simulink model "s20260831_config2torque_sim_chatgpt"  (R2025a)
settings: Solver=daessc  StartTime=0.0  StopTime=inf  FixedStep=0.01  MaxStep=0.01  RelTol=1e-3  AbsTol=1e-3  EnableMultiTasking=on
undefined symbols (not defined in the file or in its folder): X, Y, Z
libraries: sm_lib x8, nesl_utility x3, snake_single_module_library_torque x1, simulink x1, spsSawtoothGeneratorLib x1
settings Model: Creator=dperera  LastModifiedBy=dperera
settings SolverCC: AutoScaleAbsTol=off  AlgebraicLoopSolver=TrustRegion  MaxZcPerStep=1.0
settings DataIOCC: LimitDataPoints=on  MaxDataPoints=10000
settings OptimizationCC: ReuseModelBlockBuffer=off  LifeSpan=inf
settings DebuggingCC: UnconnectedInputMsg=warning  UnconnectedOutputMsg=warning  UnconnectedLineMsg=warning  AllowSymbolicDim=off  SubsystemReferenceDiagnosticForUnitTest=warning  SFUnexpectedBacktrackingDiag=warning  SFNoUnconditionalDefaultTransitionDiag=warning  SFExecutionAtInitializationDiag=none  ArithmeticOperatorsInVariantConditions=warning
settings ModelReferenceCC: EnableRefExpFcnMdlSchedulingChecks=on
settings SFSimCC: SimUseLocalCustomCode=off  CustomCodeUndefinedFunction=UseInterfaceOnly
settings RTWCC: RTWUseLocalCustomCode=off  GPUComputeCapability=3.5  DLArmComputeVersion=19.05
settings CodeAppCC: StateflowObjectComments=on
settings GRTTargetCC: TargetLangStandard=C89/C90 (ANSI)
settings ConfigComp: CovMetricSettings=dw  CovSaveCumulativeToWorkspaceVar=on  CovSaveSingleToWorkspaceVar=on  CovExternalEMLEnable=off  CovSFcnEnable=off
settings SimscapeCC: SimscapeLogType=all  SimscapeLogSimulationStatistics=on  SimscapeLogDataHistory=10000.0

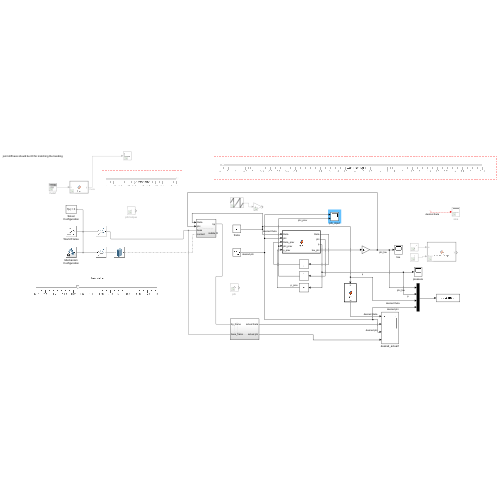
[thumbnail: Simulink's stored preview of the top-level diagram]
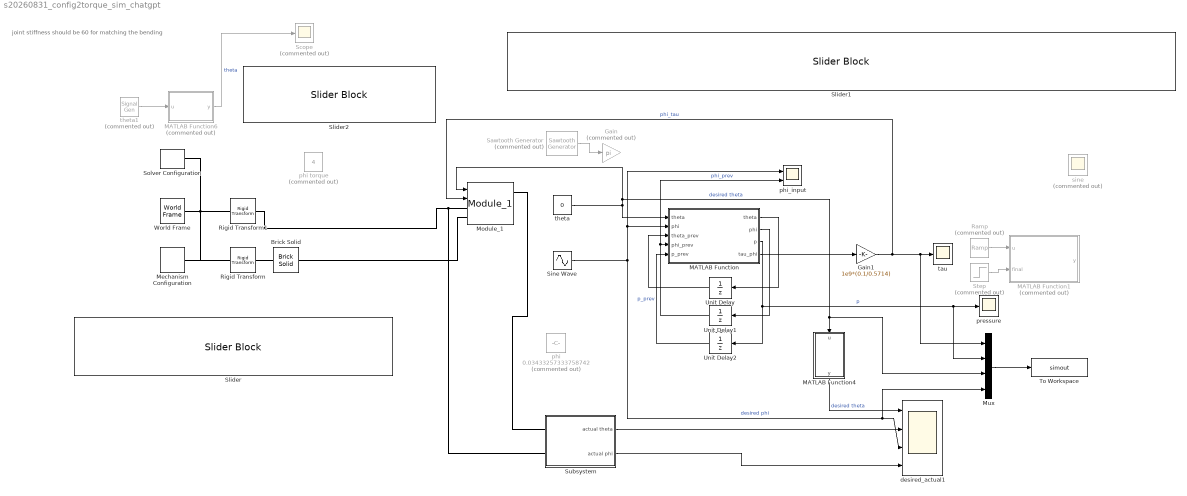
== system s20260831_config2torque_sim_chatgpt ==
  note: joint stiffness should be 60 for matching the bending
  Brick Solid : sm_lib/Body Elements/Brick Solid  BrickDimensions=[0.5 0.5 0.01]  BrickDimensionsUnits=m  ExportEntireGeometry=on  InertiaType=CalculateFromGeometry  BasedOnType=Density  Density=1000  DensityUnits=kg/m^3  Mass=1  MassUnits=kg  CenterOfMass=[0 0 0]  CenterOfMassUnits=m  MomentsOfInertia=[1 1 1]  MomentsOfInertiaUnits=kg*m^2  ProductsOfInertia=[0 0 0]  ProductsOfInertiaUnits=kg*m^2  GraphicType=FromGeometry  MarkerShape=Sphere  MarkerSize=10  GraphicVisPropType=SimpleVisualProperties  GraphicDiffuseColor=[0.5 0.5 0.5]  GraphicOpacity=1  GraphicSpecularColor=[0.5 0.5 0.5 1.0]  GraphicAmbientColor=[0.15 0.15 0.15 1.0]  GraphicEmissiveColor=[0.0 0.0 0.0 1.0]  GraphicShininess=75  DoExposeReferenceFrame=on  SerializedFrames=<Frames/>
  Gain : Gain  Commented=on  Gain=pi
  Gain1 : Gain  Gain=1e9*(0.1/0.5714)
  MATLAB Function : MATLAB Function  TreatAsAtomicUnit=on
  MATLAB Function1 : MATLAB Function  Commented=on  TreatAsAtomicUnit=on
  MATLAB Function4 : MATLAB Function  TreatAsAtomicUnit=on
  MATLAB Function6 : MATLAB Function  Commented=on  TreatAsAtomicUnit=on
  Mechanism Configuration : sm_lib/Utilities/Mechanism Configuration  UniformGravity=Constant  GravityVector=[0 0 -9.80665]  GravityVectorUnits=m/s^2  LinearizationDelta=0.001  JointModeTransitionNonlinearIterations=2
  Module_1 : snake_single_module_library_torque/Module_1  SystemSampleTime=-1  VariantActivationTime=update diagram  EmptyChoice=off  PassThrough=off  PassThroughVariantControl=(default)  EmptyChoiceVariantControl=(default)  AllowFlexibleInterface=on  Latency=0  AutoFrameSizeCalculation=off
  Mux : Mux
  Ramp : simulink/Sources/Ramp  Commented=on  slope=0.01*2*pi  start=1  InitialOutput=0.001
  Rigid Transform : sm_lib/Frames and Transforms/Rigid Transform  RotationMethod=None  FollAlignAxisA=+X  BaseAlignAxisA=+Y  FollAlignAxisB=+Y  BaseAlignAxisB=+Z  RotationStandardAxis=+Z  RotationAngle=0  RotationAngleUnits=deg  RotationArbitraryAxis=[0 0 1]  RotationSequenceAxes=FollowerAxes  RotationSequence=XYX  RotationSequenceAngles=[0 0 0]  RotationSequenceAnglesUnits=deg  RotationMatrix=[1 0 0;0 1 0;0 0 1]  Quaternion=[1 0 0 0]  TranslationMethod=StandardAxis  TranslationCartesianOffset=[0 0 0]  TranslationCartesianOffsetUnits=m  TranslationStandardAxis=+Z  TranslationStandardOffset=-0.01  TranslationStandardOffsetUnits=m  TranslationROffset=0  TranslationROffsetUnits=m  TranslationThetaOffset=0  TranslationThetaOffsetUnits=deg  TranslationZOffset=0  TranslationZOffsetUnits=m
  Rigid Transform1 : sm_lib/Frames and Transforms/Rigid Transform  RotationMethod=StandardAxis  FollAlignAxisA=+X  BaseAlignAxisA=+Y  FollAlignAxisB=+Y  BaseAlignAxisB=+Z  RotationStandardAxis=+X  RotationAngle=pi/2  RotationAngleUnits=rad  RotationArbitraryAxis=[0 0 1]  RotationSequenceAxes=FollowerAxes  RotationSequence=XYX  RotationSequenceAngles=[0 0 0]  RotationSequenceAnglesUnits=deg  RotationMatrix=[1 0 0;0 1 0;0 0 1]  Quaternion=[1 0 0 0]  TranslationMethod=None  TranslationCartesianOffset=[0 0 0]  TranslationCartesianOffsetUnits=m  TranslationStandardAxis=+Z  TranslationStandardOffset=-0.5  TranslationStandardOffsetUnits=m  TranslationROffset=0  TranslationROffsetUnits=m  TranslationThetaOffset=0  TranslationThetaOffsetUnits=deg  TranslationZOffset=0  TranslationZOffsetUnits=m
  Sawtooth Generator : spsSawtoothGeneratorLib/Sawtooth Generator  Commented=on  Freq=0.5  Phase=180  Ts=0.001
  Scope : Scope  Commented=on
      settings: ActiveDisplayYMinimum=-3.3334127281449564  ActiveDisplayYMaximum=3.1584952199962761
  Sine Wave : Sin  Amplitude=pi/2  Bias=pi/2  Phase=3*pi/2  SampleTime=0
  Slider : SliderBlock  ScaleMin=-3.14  ScaleMax=6
  Slider1 : SliderBlock  ScaleMax=3.14
  Slider2 : SliderBlock  ScaleMax=0.5
  Solver Configuration : nesl_utility/Solver Configuration  PhysicalDomain=network_engine_domain  SubClassName=solver  LeftPortType=input  RightPortType=generic  Tones=[]  Harmonics=[]  SimulateNoise=off  Profile=off  UseLocalSampling=off  EnableSwitchedLinearOptims=on  FrequencyDomain=off  UseCCode=off  RelTol=0.001  AbsTol=1e-06  MinStep=1e-09  ToWorkspace=off  RevertToSquareIcSolve=off  NumHomotopyIterations=100  PhasorMode=off  PhasorModeNumHarmonics=1  ConsistencySolver=NEWTON_XTOL_AFTER_FTOL  IndexReductionMethod=DerivativeReplacement  DoDC=off  ResidualTolerance=1e-09  ConsistencyTolSource=GLOBAL  ConsistencyAbsTol=0.001  ConsistencyRelTol=0.001  ConsistencyTolFactor=0.001  UseLocalSolver=off  LocalSolverChoice=NE_BACKWARD_EULER_ADVANCER  ResolveIndetEquations=on  FunctionEvalNumThread=1  LocalSolverSampleTime=0.001  DoFixedCost=off  MaxNonlinIter=3  MaxModeIter=2  ComputeImpulses=off  ImpulseIterations=2  LinearAlgebra=Sparse  LinearAlgebraNumThread=0  EquationFormulation=NE_TIME_EF  DelaysMemoryBudget=1024  AutomaticFiltering=on  FilteringTimeConstant=0.001  PartitionStorageMethod=AS_NEEDED  PartitionMemoryBudget=1024  PartitionMethod=FAST  MultibodyUseLocalSolver=off  MultibodyLocalSolverChoice=ODE1  MultibodyLocalSolverSampleTime=0.001
  Step : Step  Commented=on  Time=2  SampleTime=0
  Subsystem : Subsystem
  To Workspace : ToWorkspace  VariableName=simout  SaveFormat=Timeseries  SampleTime=-1
      settings: Save2DSignal=2-D array (concatenate along first dimension)
  Unit Delay : UnitDelay  InitialCondition=[0]  SampleTime=-1  HasFrameUpgradeWarning=on
  Unit Delay1 : UnitDelay  InitialCondition=0.0001  SampleTime=-1  HasFrameUpgradeWarning=on
  Unit Delay2 : UnitDelay  InitialCondition=[0.0001;0.0001;0.0001]  SampleTime=-1  HasFrameUpgradeWarning=on
  World Frame : sm_lib/Frames and Transforms/World Frame
  desired_actual1 : Scope  NumInputPorts=4
      settings: ActiveDisplayYMinimum=-0.36845329509334745  ActiveDisplayYMaximum=3.3160796558401278  DataLoggingVariableName=ScopeData7
  phi : Constant  Commented=on  Value=0.03433257333758742
  phi torque : Constant  Commented=on  Value=4
  phi_input : Scope  NumInputPorts=2
      settings: ActiveDisplayYMinimum=-0.36834079509334744  ActiveDisplayYMaximum=3.3160671558401278  DataLoggingVariableName=ScopeData3
  pressure : Scope
      settings: ActiveDisplayYMinimum=9E-5  ActiveDisplayYMaximum=0.00011  DataLoggingVariableName=ScopeData4
  sine : Scope  Commented=on
      settings: ActiveDisplayYMinimum=-0.78289652741582194  ActiveDisplayYMaximum=7.0460747695981283  DataLoggingVariableName=ScopeData2
  tau : Scope
      settings: ActiveDisplayYMinimum=-0.18280937327741567  ActiveDisplayYMaximum=1.6462948345743416
  theta : Constant  Value=0
  theta1 : SignalGenerator  Commented=on  WaveForm=sawtooth  Amplitude=pi  Frequency=0.1*2*pi  Units=rad/sec  VectorParams1D=off
  wires:
  Sawtooth Generator/1 -> Gain/1
  theta1/1 -> MATLAB Function6/1(u)
  MATLAB Function6/1(y) -> Scope/1  "theta"
  MATLAB Function/1(theta) -> Unit Delay/1
  Unit Delay/1 -> MATLAB Function/3(theta_prev)
  MATLAB Function/2(phi) -> Unit Delay1/1
  Unit Delay1/1 -> phi_input/2, MATLAB Function/4(phi_prev)  "phi_prev"
  MATLAB Function/3(p) -> Unit Delay2/1, Mux/2, pressure/1  "p"
  Unit Delay2/1 -> MATLAB Function/5(p_prev)  "p_prev"
  theta/1 -> MATLAB Function/1("theta "), Module_1/1, Mux/3, MATLAB Function4/1(u)  "desired theta"
  MATLAB Function/4(tau_phi) -> Gain1/1
  Ramp/1 -> MATLAB Function1/1(u)
  Step/1 -> MATLAB Function1/2(final)
  MATLAB Function4/1(y) -> desired_actual1/1  "desired theta"
  Gain1/1 -> Module_1/2, Mux/1, tau/1  "phi_tau"
  Sine Wave/1 -> phi_input/1, MATLAB Function/2("phi "), Mux/4, desired_actual1/3  "desired phi"
  Subsystem/1(actual theta) -> desired_actual1/2
  Subsystem/2(actual phi) -> desired_actual1/4
  Mux/1 -> To Workspace/1
  ? -> sine/1  "desired theta"
  connections:
  World Frame/RConn1 -- Rigid Transform/LConn1 -- Mechanism Configuration/RConn1 -- Rigid Transform1/LConn1 -- Solver Configuration/RConn1
  Brick Solid/RConn1 -- Rigid Transform/RConn1
  Module_1/LConn1 -- Rigid Transform1/RConn1 -- Subsystem/LConn2
  Brick Solid/LConn1 -- Module_1/LConn2
  Subsystem/LConn1 -- Module_1/RConn1

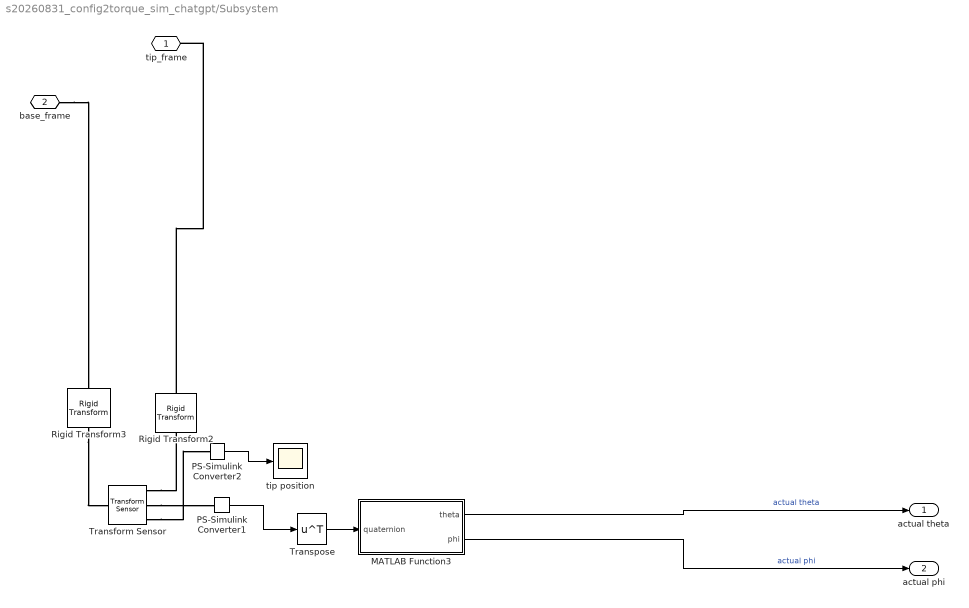
== system s20260831_config2torque_sim_chatgpt/Subsystem ==
  MATLAB Function3 : MATLAB Function  TreatAsAtomicUnit=on
  PS-Simulink Converter1 : nesl_utility/PS-Simulink Converter  PhysicalDomain=network_engine_domain  SubClassName=ps_output  LeftPortType=input  RightPortType=output  PseudoPeriodic=off  Frequencies=[]  VectorFormat=inherit  Unit=inherit  AffineConversion=off
  PS-Simulink Converter2 : nesl_utility/PS-Simulink Converter  PhysicalDomain=network_engine_domain  SubClassName=ps_output  LeftPortType=input  RightPortType=output  PseudoPeriodic=off  Frequencies=[]  VectorFormat=inherit  Unit=inherit  AffineConversion=off
  Rigid Transform2 : sm_lib/Frames and Transforms/Rigid Transform  RotationMethod=RotationSequence  FollAlignAxisA=+X  BaseAlignAxisA=+Y  FollAlignAxisB=+Y  BaseAlignAxisB=+Z  RotationStandardAxis=+Z  RotationAngle=pi  RotationAngleUnits=rad  RotationArbitraryAxis=[0 0 1]  RotationSequenceAxes=FollowerAxes  RotationSequence=XZY  RotationSequenceAngles=[-pi/2 pi 0]  RotationSequenceAnglesUnits=rad  RotationMatrix=[1 0 0;0 1 0;0 0 1]  Quaternion=[1 0 0 0]  TranslationMethod=None  TranslationCartesianOffset=[0 0 0]  TranslationCartesianOffsetUnits=m  TranslationStandardAxis=+Z  TranslationStandardOffset=-0.5  TranslationStandardOffsetUnits=m  TranslationROffset=0  TranslationROffsetUnits=m  TranslationThetaOffset=0  TranslationThetaOffsetUnits=deg  TranslationZOffset=0  TranslationZOffsetUnits=m
  Rigid Transform3 : sm_lib/Frames and Transforms/Rigid Transform  RotationMethod=RotationSequence  FollAlignAxisA=+X  BaseAlignAxisA=+Y  FollAlignAxisB=+Y  BaseAlignAxisB=+Z  RotationStandardAxis=+Z  RotationAngle=pi  RotationAngleUnits=rad  RotationArbitraryAxis=[0 0 1]  RotationSequenceAxes=FollowerAxes  RotationSequence=YXZ  RotationSequenceAngles=[pi -pi/2 0]  RotationSequenceAnglesUnits=rad  RotationMatrix=[1 0 0;0 1 0;0 0 1]  Quaternion=[1 0 0 0]  TranslationMethod=None  TranslationCartesianOffset=[0 0 0]  TranslationCartesianOffsetUnits=m  TranslationStandardAxis=+Z  TranslationStandardOffset=-0.5  TranslationStandardOffsetUnits=m  TranslationROffset=0  TranslationROffsetUnits=m  TranslationThetaOffset=0  TranslationThetaOffsetUnits=deg  TranslationZOffset=0  TranslationZOffsetUnits=m
  Transform Sensor : sm_lib/Frames and Transforms/Transform Sensor  MeasurementFrame=Follower  RotationSequence=XYZ  SenseAngle=off  SenseAxis=off  SenseQ=on  SenseR=off  SenseRotationSequence=off  SenseOmegaX=off  SenseOmegaY=off  SenseOmegaZ=off  SenseOmega=off  SenseQDot=off  SenseRDot=off  SenseRotationSequenceDot=off  SenseAlphaX=off  SenseAlphaY=off  SenseAlphaZ=off  SenseAlpha=off  SenseQDDot=off  SenseRDDot=off  SenseX=off  SenseY=off  SenseZ=off  SenseXYZ=on  SenseRad=off  SenseAzim=off  SenseDist=off  SenseInc=off  SenseXDot=off  SenseYDot=off  SenseZDot=off  SenseXYZDot=off  SenseRadDot=off  SenseAzimDot=off  SenseDistDot=off  SenseIncDot=off  SenseXDDot=off  SenseYDDot=off  SenseZDDot=off  SenseXYZDDot=off  SenseRadDDot=off  SenseAzimDDot=off  SenseDistDDot=off  SenseIncDDot=off
  Transpose : Math  Operator=transpose
  tip position : Scope
      settings: ActiveDisplayYMinimum=-0.036250000065594909  ActiveDisplayYMaximum=0.32625000000729432  DataLoggingVariableName=ScopeData6
  tip_frame : PMIOPort  Side=Left
  base_frame : PMIOPort  Port=2  Side=Left
  actual theta : Outport
  actual phi : Outport  Port=2
  wires:
  PS-Simulink Converter1/1 -> Transpose/1
  Transpose/1 -> MATLAB Function3/1(quaternion)
  MATLAB Function3/2(phi) -> actual phi/1  "actual phi"
  PS-Simulink Converter2/1 -> tip position/1
  MATLAB Function3/1(theta) -> actual theta/1  "actual theta"
  connections:
  Transform Sensor/RConn1 -- Rigid Transform2/RConn1
  Transform Sensor/RConn2 -- PS-Simulink Converter1/LConn1
  Rigid Transform3/RConn1 -- Transform Sensor/LConn1
  Transform Sensor/RConn3 -- PS-Simulink Converter2/LConn1
  base_frame/RConn1 -- Rigid Transform3/LConn1
  Rigid Transform2/LConn1 -- tip_frame/RConn1

== matlab function s20260831_config2torque_sim_chatgpt/MATLAB Function1 ==
  data: u input; y output; final input
function y = smoothStep(u, final)

y = u*(1-final);

if y <= 0.00001
    y= 0.001;
end

end

== matlab function s20260831_config2torque_sim_chatgpt/MATLAB Function ==
  data: theta input; theta output; phi input; theta_prev input; phi_prev input; p_prev input; phi output; p output; tau_phi output
function [theta, phi, p, tau_phi] = fcn(theta, phi, theta_prev, phi_prev, p_prev)
%#codegen 
% 
% This function computes torque required for the
% 
A = pi * (0.013/2)^2;
r = 0.013;
K = 0.00001;
N = 30;
L = 0.29;
l = L/N;

J_angle = f20260427_3_pressure2config_Jacobian(p_prev, A, K, r);
J_inv = pinv(J_angle);
% p = p_mat(:, i) + J_inv*([theta(i+1); phi(i+1)]-[frw(1,i); frw(2,i)]);
p = p_prev + J_inv*([theta; phi]-[theta_prev; phi_prev]);
% p = m20260427_5_PositivePressures(p);


[f, my, mx, ~, ~] = pressure2force_moment_config(p, A, r, K);
W = [mx; my; 0.0; 0.0; 0.0; f];
J = completeArm_Jacobian(theta_prev, phi_prev, l, N);

tau = J' * W;
tau_phi = tau(2);

== matlab function s20260831_config2torque_sim_chatgpt/Subsystem/MATLAB Function3 ==
  data: quaternion input; theta output; phi output
function [theta, phi] = IMU2Config(quaternion)
%#codegen
T = quat2rotm(quaternion);

theta= wrapToPi(atan2(T(2,3),T(1,3)));
phi= (acos(T(3,3)));

end

== matlab function s20260831_config2torque_sim_chatgpt/MATLAB Function4 ==
  data: u input; y output
function y = fcn(u)
%$codegen
y = wrapToPi(u);

== matlab function s20260831_config2torque_sim_chatgpt/MATLAB Function6 ==
  data: u input; y output
function y = fcn(u)

y = wrapToPi(u - pi);
